simulink model "Simulation"  (R2016a)
settings: Solver=FixedStepAuto  StartTime=0.0  StopTime=100  RelTol=1e-3
undefined symbols (not defined in the file): A, B, C, D, Discrete, R, Time
libraries: dspstat3 x2, ctrlSharedLib x1, neural x1
settings Model: Creator=geraw  LastModifiedBy=geraw

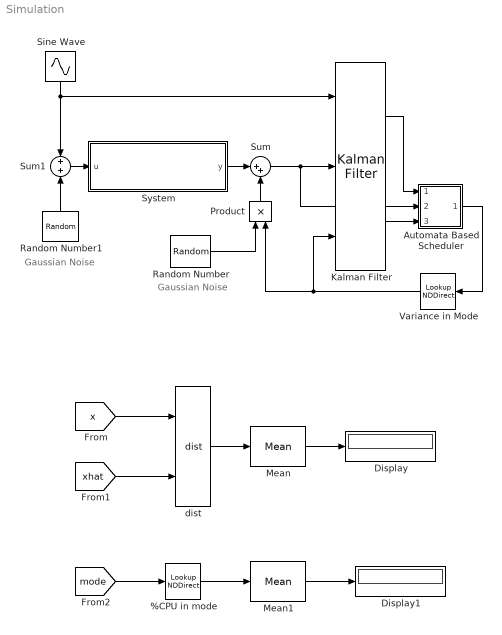
== system Simulation ==
  note: Gaussian Noise
  note: Gaussian Noise
  %CPU in mode : LookupNDDirect  NumberOfTableDimensions=1  Table=[1.1-0.25;1.1-1]
  Automata Based Scheduler : Subsystem
      mask Display: image('C:\Users\geraw\Dropbox\Papers\ICCPS_2018_Hodai\automaton.png');
  Display : Display
  Display1 : Display
  Kalman Filter : ctrlSharedLib/Kalman Filter  TimeDomain=Discrete-Time  UseCurrentEstimator=off  ModelSource=Individual A, B, C, D matrices  ModelSourceVariable=sys  A=A  B=B  C=C  D=D  NumberOfStates=2  NumberOfInputs=2  NumberOfOutputs=2  InitialEstimateSource=Dialog  X0=0  P0=5  UseK=off  UseGH=on  NumberOfProcessNoiseInputs=2  G=B  TimeInvariantG=on  H=0  TimeInvariantH=on  Q=1  TimeInvariantQ=on  R=R  TimeInvariantR=off  N=0  TimeInvariantN=on  AddInputPort=on  AddEnablePort=off  OutputEstimatedY=on  OutputP=off  Ts=1
  Mean : dspstat3/Mean  run=on  reset_popup=None  InputProcessing=Columns as channels (frame based)  directionMode=Each column  dimension=1  roiEnable=off  roiType=Rectangles  roiPortion=Entire ROI  roiOutput=Individual statistics for each ROI  roiFlag=off  outputDataTypeStr=Inherit: Same as accumulator  outputLastDataTypeStr=Inherit: Same as accumulator  outputMin=[]  outputMax=[]  roundingMode=Floor  overflowMode=off
  Mean1 : dspstat3/Mean  run=on  reset_popup=None  InputProcessing=Columns as channels (frame based)  directionMode=Each column  dimension=1  roiEnable=off  roiType=Rectangles  roiPortion=Entire ROI  roiOutput=Individual statistics for each ROI  roiFlag=off  outputDataTypeStr=Inherit: Same as accumulator  outputLastDataTypeStr=Inherit: Same as accumulator  outputMin=[]  outputMax=[]  roundingMode=Floor  overflowMode=off
  Product : Product
  Random Number : RandomNumber  SampleTime=1
  Random Number1 : RandomNumber  SampleTime=1
  Sine Wave : Sin  Bias=1  SampleTime=1
  Sum : Sum  Inputs=|++
  Sum1 : Sum
  "System " : Subsystem
      mask Display: image('C:\Users\geraw\Dropbox\Papers\ICCPS_2018_Hodai\LTI.JPG');
  Variance in Mode : LookupNDDirect  NumberOfTableDimensions=1  Table=[0.25;1]
  dist : neural/Weight Functions/dist
  wires:
  Sum/1 -> Automata Based Scheduler/2(In1), Kalman Filter/2
  Sum1/1 -> "System "/1(u)
  "System "/1(y) -> Sum/1
  Product/1 -> Sum/2
  Random Number/1 -> Product/1
  Random Number1/1 -> Sum1/2
  Sine Wave/1 -> Sum1/1, Kalman Filter/1
  Kalman Filter/2 -> Automata Based Scheduler/3(In2)
  Automata Based Scheduler/1(Out1) -> Variance in Mode/1
  Kalman Filter/1 -> Automata Based Scheduler/1(In3)
  Variance in Mode/1 -> Product/2, Kalman Filter/3
  [x] -> dist/1
  [xhat] -> dist/2
  dist/1 -> Mean/1
  Mean/1 -> Display/1
  [mode] -> %CPU in mode/1
  %CPU in mode/1 -> Mean1/1
  Mean1/1 -> Display1/1

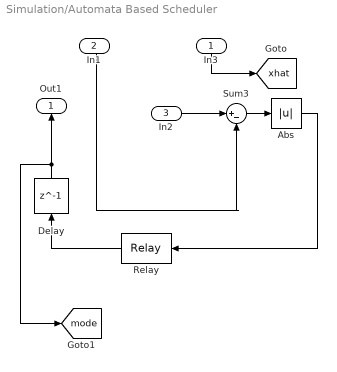
== system Simulation/Automata Based Scheduler ==
  In3 : Inport
  In1 : Inport  Port=2
  In2 : Inport  Port=3
  Abs : Abs
  Delay : Delay  DelayLength=1  InitialCondition=0.25
  Relay : Relay  OnSwitchValue=1  OffSwitchValue=0.5  OnOutputValue=0  OffOutputValue=1  InputProcessing=Columns as channels (frame based)
  Sum3 : Sum  Inputs=|+-
  Out1 : Outport
  tag scope: mode=global, xhat=global
  wires:
  Delay/1 -> Out1/1, [mode]
  Relay/1 -> Delay/1
  In2/1 -> Sum3/1
  Sum3/1 -> Abs/1
  In1/1 -> Sum3/2
  Abs/1 -> Relay/1
  In3/1 -> [xhat]

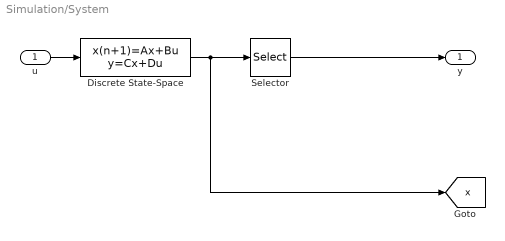
== system Simulation/System  ==
  u : Inport
  Discrete State-Space : DiscreteStateSpace  A=A  B=B  C=eye(3)  D=[0; 0; 0]  X0=[1;2;3]  StateIdentifier=x
  Selector : Selector  InputPortWidth=3  IndexOptions=Index vector (dialog)  Indices=[1]  OutputSizes=1
  y : Outport
  tag scope: x=global
  wires:
  Discrete State-Space/1 -> [x], Selector/1
  u/1 -> Discrete State-Space/1
  Selector/1 -> y/1
